simulink subsystem "Mq_SubSystem"  (R2020b)
settings: Solver=VariableStepAuto  StartTime=0.0  StopTime=10.0  RelTol=1e-3
values from neighbouring files (symbols this model uses):
  Irotyy = mot.rot.Iyy    [Electromechanical.m]
  l = body.zb    [Electromechanical.m]
  M11q = 2*Iwyy + 2*Irotyy*n^2 + (mb + 2*(mrot+mw))*r^2    [Electromechanical.m]
  M22q = Ibyy + 2*(1-n)^2*Irotyy + mb*l^2 + 2*mrot*zbrot^2    [Electromechanical.m]
  mb = body.m    [Electromechanical.m]
  mrot = mot.rot.m    [Electromechanical.m]
  n = gbox.N    [Electromechanical.m]
  r = wheel.r    [Electromechanical.m]
  Ts = 1e-2    (= 0.01)    [balrob_params.m]
  zbrot = mot.rot.zb    [Electromechanical.m]
settings Model: Creator=umberto  LastModifiedBy=umberto

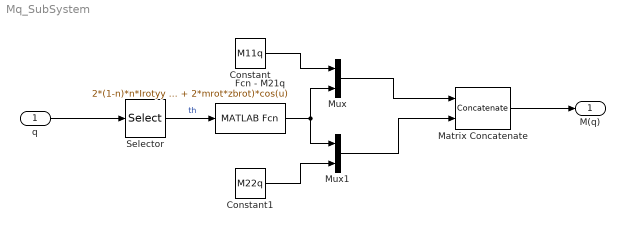
== system Mq_SubSystem ==
  q : Inport
  Constant : Constant  Value=M11q  SampleTime=Ts
  Constant1 : Constant  Value=M22q  SampleTime=Ts
  Fcn - M21q : MATLABFcn  MATLABFcn=2*(1-n)*n*Irotyy + r*(l*mb + 2*mrot*zbrot)*cos(u)
  Matrix Concatenate : Concatenate  Mode=Multidimensional array  ConcatenateDimension=2
  Mux : Mux  Inputs=2
  Mux1 : Mux  Inputs=2
  Selector : Selector  InputPortWidth=2  IndexOptions=Index vector (dialog)  Indices=[2]  OutputSizes=1
  M(q) : Outport
  wires:
  q/1 -> Selector/1
  Selector/1 -> Fcn - M21q/1  "th"
  Fcn - M21q/1 -> Mux/2, Mux1/1
  Constant1/1 -> Mux1/2
  Constant/1 -> Mux/1
  Mux/1 -> Matrix Concatenate/1
  Mux1/1 -> Matrix Concatenate/2
  Matrix Concatenate/1 -> M(q)/1
